simulink model "ThdRwRtStFwdBkwdHolderChk"  (R2018b)
settings: Solver=FixedStepDiscrete  StartTime=0.0  StopTime=10.0  FixedStep=0.01  RelTol=1e-3
libraries: simulink x2
settings Model: Creator=sn2xws  LastModifiedBy=sn2xws
settings Model: ModifiedHistory=|
  | V2.2.0 557 模式流程V1.6
  | V3.0.0 retry信号连线遗漏
  | 25.7.4 V3.13.0 新增Md61 Md62
settings DataIOCC: SaveFormat=StructureWithTime
settings OptimizationCC: DefaultParameterBehavior=Inlined  EnhancedBackFolding=on  PassReuseOutputArgsAs=Individual arguments  ZeroExternalMemoryAtStartup=off  ZeroInternalMemoryAtStartup=off  OptimizeBlockOrder=speed  DifferentSizesBufferReuse=on  OptimizationCustomize=off
settings DebuggingCC: ParameterTunabilityLossMsg=error
settings ModelReferenceCC: ModelReferenceNumInstancesAllowed=Single
settings SFSimCC: MATLABDynamicMemAlloc=off
settings RTWCC: SystemTargetFile=autosar.tlc  GenCodeOnly=on  TemplateMakefile=ert_default_tmf  Description=AUTOSAR  GenerateReport=on  IncludeHyperlinkInReport=on  LaunchReport=on  GenerateTraceInfo=on  GenerateTraceReport=on  GenerateTraceReportSl=on  GenerateTraceReportSf=on  GenerateTraceReportEml=on
settings CodeAppCC: ForceParamTrailComments=on  IgnoreCustomStorageClasses=off  OperatorAnnotations=on  SimulinkDataObjDesc=on  SFDataObjDesc=on  InsertBlockDesc=on
settings STFCustomTargetCC: TargetLangStandard=C99 (ISO)  MultiwordLength=256  ParMdlRefBuildCompliant=on  CompOptLevelCompliant=on  IncludeMdlTerminateFcn=off  CombineOutputUpdateFcns=on  SuppressErrorStatus=on  ERTCustomFileBanners=on  SupportNonFinite=off  SupportComplex=off  SupportContinuousTime=off  SupportNonInlinedSFcns=off  RemoveResetFunc=on  MATLABClassNameForMDSCustomization=Simulink.SoftwareTarget.ERTCustomization  AutosarCompliant=on  UseToolchainInfoCompliant=on  LookupTableObjectStructAxisOrder=2,1,3,4,...  LUTObjectStructOrderEvenSpacing=Size,Table,Breakpoints  SystemTargetFile=autosar.tlc
settings ERTTargetCC: TargetLangStandard=C99 (ISO)  ConcurrentExecutionCompliant=off  IncludeMdlTerminateFcn=off  SuppressErrorStatus=on  SupportNonFinite=off  SupportComplex=off  ModelStepFunctionPrototypeControlCompliant=off  CPPClassGenCompliant=off  AutosarCompliant=on  LookupTableObjectStructAxisOrder=2,1,3,4,...  LUTObjectStructOrderEvenSpacing=Size,Table,Breakpoints  InlinedParameterPlacement=NonHierarchical  ERTCustomFileTemplate=example_file_process.tlc  ERTFilePackagingFormat=Compact

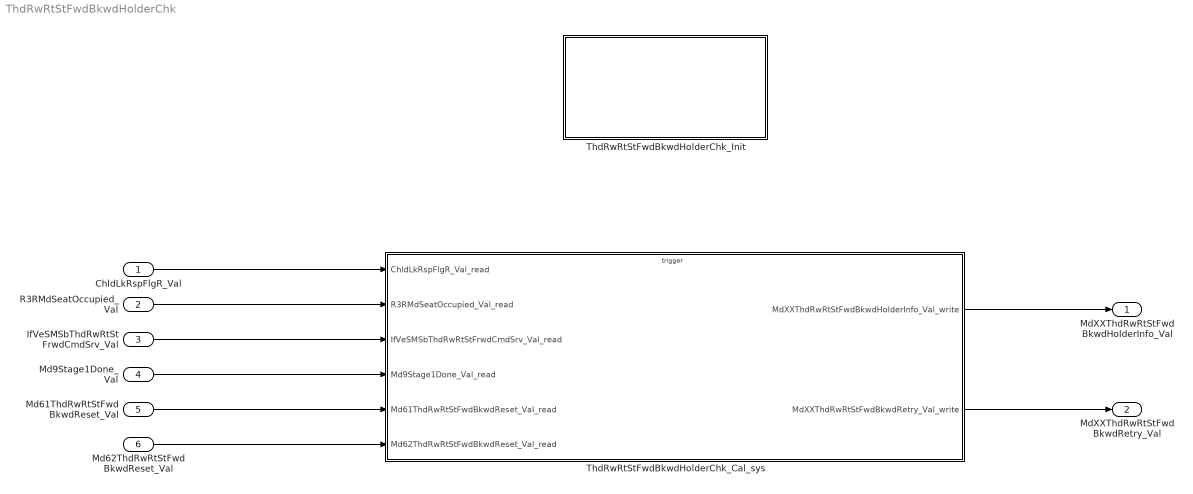
== system ThdRwRtStFwdBkwdHolderChk ==
  ChldLkRspFlgR_Val : Inport  OutDataTypeStr=boolean  PortDimensions=1
  R3RMdSeatOccupied_Val : Inport  Port=2  OutDataTypeStr=boolean  PortDimensions=1
  IfVeSMSbThdRwRtStFrwdCmdSrv_Val : Inport  Port=3  OutDataTypeStr=boolean  PortDimensions=1
  Md9Stage1Done_Val : Inport  Port=4  OutDataTypeStr=boolean  PortDimensions=1
  Md61ThdRwRtStFwdBkwdReset_Val : Inport  Port=5  OutDataTypeStr=boolean  PortDimensions=1
  Md62ThdRwRtStFwdBkwdReset_Val : Inport  Port=6  OutDataTypeStr=boolean  PortDimensions=1
  ThdRwRtStFwdBkwdHolderChk_Cal_sys : Subsystem
  ThdRwRtStFwdBkwdHolderChk_Init : Subsystem
  MdXXThdRwRtStFwdBkwdHolderInfo_Val : Outport  OutDataTypeStr=uint32  PortDimensions=1
  MdXXThdRwRtStFwdBkwdRetry_Val : Outport  Port=2  OutDataTypeStr=uint32  PortDimensions=1
  wires:
  ChldLkRspFlgR_Val/1 -> ThdRwRtStFwdBkwdHolderChk_Cal_sys/1(ChldLkRspFlgR_Val_read)
  R3RMdSeatOccupied_Val/1 -> ThdRwRtStFwdBkwdHolderChk_Cal_sys/2(R3RMdSeatOccupied_Val_read)
  ThdRwRtStFwdBkwdHolderChk_Cal_sys/1(MdXXThdRwRtStFwdBkwdHolderInfo_Val_write) -> MdXXThdRwRtStFwdBkwdHolderInfo_Val/1
  IfVeSMSbThdRwRtStFrwdCmdSrv_Val/1 -> ThdRwRtStFwdBkwdHolderChk_Cal_sys/3(IfVeSMSbThdRwRtStFrwdCmdSrv_Val_read)
  Md9Stage1Done_Val/1 -> ThdRwRtStFwdBkwdHolderChk_Cal_sys/4(Md9Stage1Done_Val_read)
  ThdRwRtStFwdBkwdHolderChk_Cal_sys/2(MdXXThdRwRtStFwdBkwdRetry_Val_write) -> MdXXThdRwRtStFwdBkwdRetry_Val/1
  Md61ThdRwRtStFwdBkwdReset_Val/1 -> ThdRwRtStFwdBkwdHolderChk_Cal_sys/5(Md61ThdRwRtStFwdBkwdReset_Val_read)
  Md62ThdRwRtStFwdBkwdReset_Val/1 -> ThdRwRtStFwdBkwdHolderChk_Cal_sys/6(Md62ThdRwRtStFwdBkwdReset_Val_read)

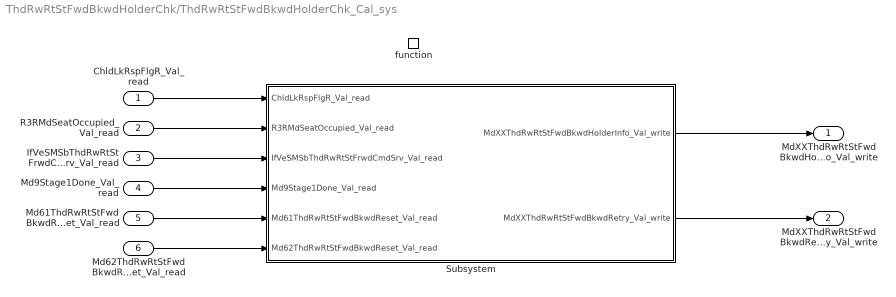
== system ThdRwRtStFwdBkwdHolderChk/ThdRwRtStFwdBkwdHolderChk_Cal_sys ==
  ChldLkRspFlgR_Val_read : Inport
  R3RMdSeatOccupied_Val_read : Inport  Port=2
  IfVeSMSbThdRwRtStFrwdCmdSrv_Val_read : Inport  Port=3
  Md9Stage1Done_Val_read : Inport  Port=4
  Md61ThdRwRtStFwdBkwdReset_Val_read : Inport  Port=5
  Md62ThdRwRtStFwdBkwdReset_Val_read : Inport  Port=6
  function : TriggerPort  TriggerType=function-call  IsSimulinkFunction=on  FunctionName=ThdRwRtStFwdBkwdHolderChk_Cal  VariantControl=(inherit)
  Subsystem : Subsystem
  MdXXThdRwRtStFwdBkwdHolderInfo_Val_write : Outport
      settings: EnsureOutportIsVirtual=on
  MdXXThdRwRtStFwdBkwdRetry_Val_write : Outport  Port=2
      settings: EnsureOutportIsVirtual=on
  wires:
  ChldLkRspFlgR_Val_read/1 -> Subsystem/1(ChldLkRspFlgR_Val_read)
  R3RMdSeatOccupied_Val_read/1 -> Subsystem/2(R3RMdSeatOccupied_Val_read)
  Subsystem/1(MdXXThdRwRtStFwdBkwdHolderInfo_Val_write) -> MdXXThdRwRtStFwdBkwdHolderInfo_Val_write/1
  IfVeSMSbThdRwRtStFrwdCmdSrv_Val_read/1 -> Subsystem/3(IfVeSMSbThdRwRtStFrwdCmdSrv_Val_read)
  Md9Stage1Done_Val_read/1 -> Subsystem/4(Md9Stage1Done_Val_read)
  Subsystem/2(MdXXThdRwRtStFwdBkwdRetry_Val_write) -> MdXXThdRwRtStFwdBkwdRetry_Val_write/1
  Md61ThdRwRtStFwdBkwdReset_Val_read/1 -> Subsystem/5(Md61ThdRwRtStFwdBkwdReset_Val_read)
  Md62ThdRwRtStFwdBkwdReset_Val_read/1 -> Subsystem/6(Md62ThdRwRtStFwdBkwdReset_Val_read)

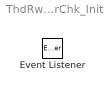
== system ThdRwRtStFwdBkwdHolderChk/ThdRwRtStFwdBkwdHolderChk_Init ==
  Event Listener : EventListener  EventName=reset

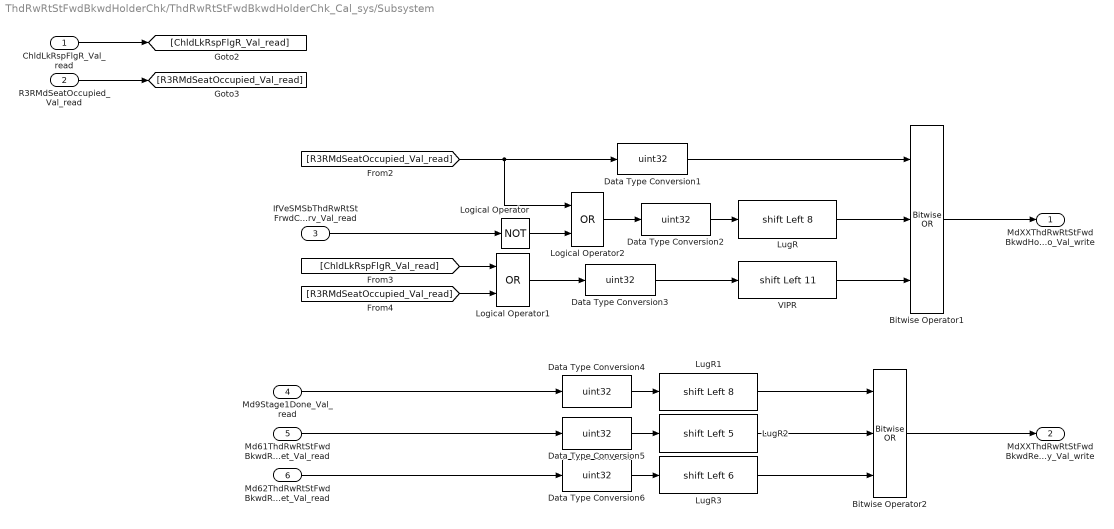
== system ThdRwRtStFwdBkwdHolderChk/ThdRwRtStFwdBkwdHolderChk_Cal_sys/Subsystem ==
  ChldLkRspFlgR_Val_read : Inport
  R3RMdSeatOccupied_Val_read : Inport  Port=2
  IfVeSMSbThdRwRtStFrwdCmdSrv_Val_read : Inport  Port=3
  Md9Stage1Done_Val_read : Inport  Port=4
  Md61ThdRwRtStFwdBkwdReset_Val_read : Inport  Port=5
  Md62ThdRwRtStFwdBkwdReset_Val_read : Inport  Port=6
  Bitwise Operator1 : simulink/Logic and Bit Operations/Bitwise Operator  logicop=OR  UseBitMask=off  NumInputPorts=3  BitMask=bin2dec('11011001')  BitMaskRealWorld=Stored Integer
  Bitwise Operator2 : simulink/Logic and Bit Operations/Bitwise Operator  logicop=OR  UseBitMask=off  NumInputPorts=3  BitMask=bin2dec('11011001')  BitMaskRealWorld=Stored Integer
  Data Type Conversion{1..6} (6 alike) : DataTypeConversion  OutDataTypeStr=uint32
  Logical Operator : Logic  Operator=NOT  AllPortsSameDT=off  OutDataTypeStr=boolean
  Logical Operator1 : Logic  Operator=OR  AllPortsSameDT=off  OutDataTypeStr=boolean
  Logical Operator2 : Logic  Operator=OR  AllPortsSameDT=off  OutDataTypeStr=boolean
  LugR : ArithShift  BitShiftNumber=8  BitShiftDirection=Left
  LugR1 : ArithShift  BitShiftNumber=8  BitShiftDirection=Left
  LugR2 : ArithShift  BitShiftNumber=5  BitShiftDirection=Left
  LugR3 : ArithShift  BitShiftNumber=6  BitShiftDirection=Left
  VIPR : ArithShift  BitShiftNumber=11  BitShiftDirection=Left
  MdXXThdRwRtStFwdBkwdHolderInfo_Val_write : Outport
      settings: EnsureOutportIsVirtual=on
  MdXXThdRwRtStFwdBkwdRetry_Val_write : Outport  Port=2
      settings: EnsureOutportIsVirtual=on
  wires:
  Bitwise Operator1/1 -> MdXXThdRwRtStFwdBkwdHolderInfo_Val_write/1
  [ChldLkRspFlgR_Val_read] -> Logical Operator1/1
  Data Type Conversion3/1 -> VIPR/1
  [R3RMdSeatOccupied_Val_read] -> Logical Operator1/2
  Data Type Conversion1/1 -> Bitwise Operator1/1
  ChldLkRspFlgR_Val_read/1 -> [ChldLkRspFlgR_Val_read]
  Logical Operator1/1 -> Data Type Conversion3/1
  LugR/1 -> Bitwise Operator1/2
  VIPR/1 -> Bitwise Operator1/3
  [R3RMdSeatOccupied_Val_read] -> Logical Operator2/1, Data Type Conversion1/1
  R3RMdSeatOccupied_Val_read/1 -> [R3RMdSeatOccupied_Val_read]
  IfVeSMSbThdRwRtStFrwdCmdSrv_Val_read/1 -> Logical Operator/1
  Logical Operator/1 -> Logical Operator2/2
  Data Type Conversion2/1 -> LugR/1
  Logical Operator2/1 -> Data Type Conversion2/1
  Md9Stage1Done_Val_read/1 -> Data Type Conversion4/1
  Data Type Conversion4/1 -> LugR1/1
  Data Type Conversion5/1 -> LugR2/1
  Md61ThdRwRtStFwdBkwdReset_Val_read/1 -> Data Type Conversion5/1
  Md62ThdRwRtStFwdBkwdReset_Val_read/1 -> Data Type Conversion6/1
  Data Type Conversion6/1 -> LugR3/1
  LugR1/1 -> Bitwise Operator2/1
  LugR2/1 -> Bitwise Operator2/2
  LugR3/1 -> Bitwise Operator2/3
  Bitwise Operator2/1 -> MdXXThdRwRtStFwdBkwdRetry_Val_write/1
